simulink model "motor_m_china"  (R2022a)
settings: Solver=VariableStepAuto  StartTime=0.0  StopTime=10.0  RelTol=1e-3
undefined symbols (not defined in the file): B, J, ke, kt, L, R
settings Model: Creator=farfar  LastModifiedBy=farfar

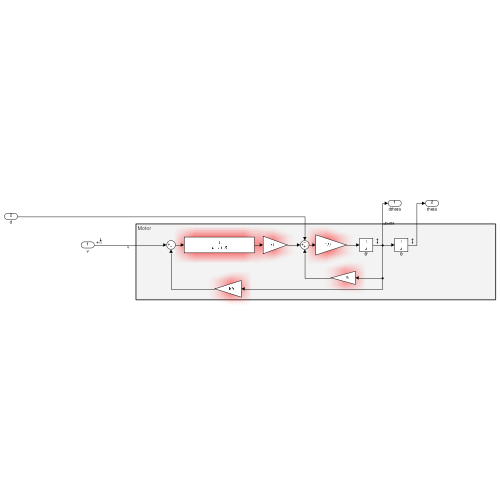
[thumbnail: Simulink's stored preview of the top-level diagram]
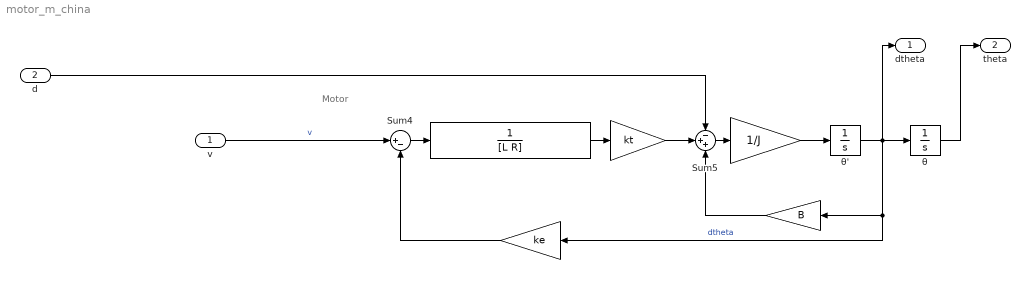
== system motor_m_china ==
  note: Motor
  v : Inport
  d : Inport  Port=2
  " " : Gain  Gain=1/J
  "  " : Gain  Gain=B
  "   " : Gain  Gain=ke
  "    " : TransferFcn  Denominator=[L R]
  "     " : Gain  Gain=kt
  Sum4 : Sum  Inputs=|+-
  Sum5 : Sum  Inputs=-++
  θ : Integrator
  θ' : Integrator
  dtheta : Outport
  theta : Outport  Port=2
  wires:
  "  "/1 -> Sum5/3
  " "/1 -> θ'/1
  "    "/1 -> "     "/1
  d/1 -> Sum5/1
  Sum4/1 -> "    "/1
  v/1 -> Sum4/1  "v"
  θ'/1 -> dtheta/1, θ/1, "  "/1, "   "/1  "dtheta"
  "   "/1 -> Sum4/2
  Sum5/1 -> " "/1
  "     "/1 -> Sum5/2
  θ/1 -> theta/1
